simulink model "new"  (R2020b)
settings: Solver=VariableStepAuto  StartTime=0.0  StopTime=1  RelTol=1e-3
settings Model: Creator=99003778  LastModifiedBy=99003778

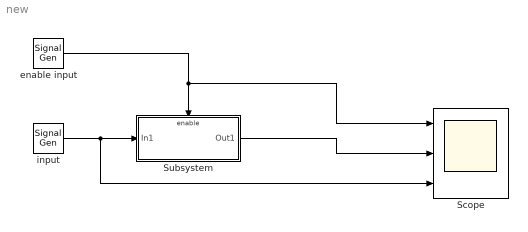
== system new ==
  Scope : Scope  NumInputPorts=3
  Subsystem : Subsystem
  enable input : SignalGenerator  WaveForm=square
  input : SignalGenerator
  wires:
  input/1 -> Scope/3, Subsystem/1(In1)
  enable input/1 -> Scope/1, Subsystem/Enable
  Subsystem/1(Out1) -> Scope/2

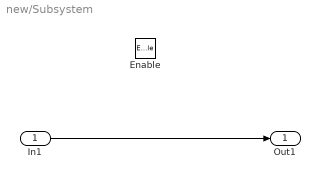
== system new/Subsystem ==
  In1 : Inport
  Enable : EnablePort
  Out1 : Outport
  wires:
  In1/1 -> Out1/1
